simulink model "Powertrain"  (R2020a)
settings: Solver=VariableStepAuto  StartTime=0.0  StopTime=10.0  RelTol=1e-3
values from neighbouring files (symbols this model uses):
  lambda_pm = 0.1194    [MotGenEvDynamicDD.sldd]
undefined symbols (not defined in the file or in its folder): DiscIntNeverNeededParam, Ion, Lithium
libraries: powerlib x12, electricdrivelib x2, powerlib_meascontrol x2, autolibdatasheetbattery x1, simulink x1, autolibmotorctrlr x1, autolibpmsminterior x1, autolibinverter x1
settings Model: Creator=Ricky  LastModifiedBy=Ricky

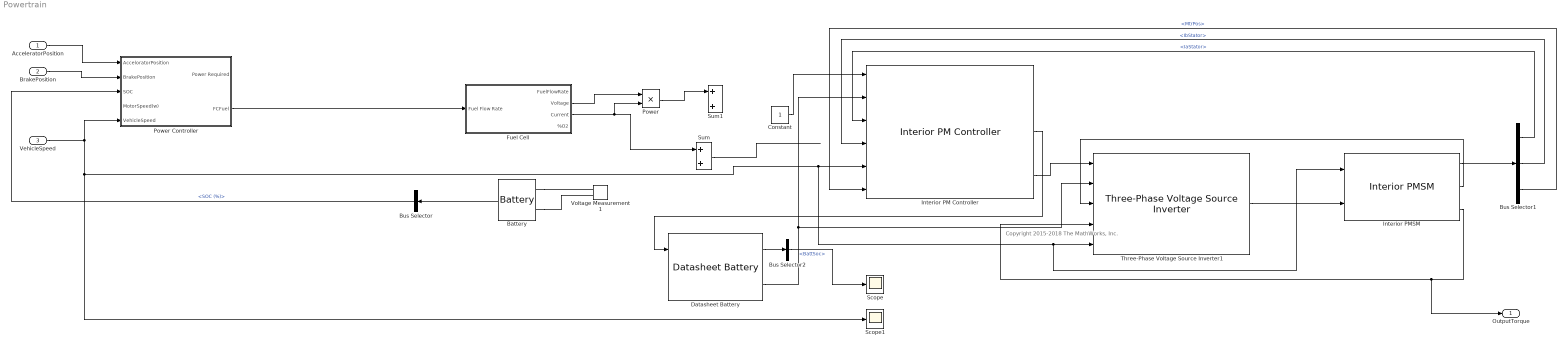
== system Powertrain ==
  note: Copyright 2015-2018 The MathWorks, Inc.
  AcceleratorPosition : Inport
  BrakePosition : Inport  Port=2
  VehicleSpeed : Inport  Port=3
  Battery : electricdrivelib/Extra Sources/Battery  BatType=Lithium-Ion  ShowTempParam=off  ThermalPreset=no  ShowAgeParam=off  NomV=7.2  NomQ=5.4  SOC=100  Batt_Tr=30  PresetModel=on  MaxQ=5.4  MinV=5.4  FullV=8.3807  Dis_rate=2.3478  R=0.013333  Normal_OP=4.8835  expZone="[7.7788      0.2653]"  current=[6.5 13 32.5]  Units=Time  Tci=20  NomT=20  T2=-30  MaxQ2=4.8  FullV2=7.1  Normal_OP2=5.655  expZone2="[6.58           1]"  Rca=0.6  ti=2000  Dp=0  Neq0=0  Tsim=1e6  Ta1=25  Qeol=5.4*0.9  Reol=0.013333*1.2  Char_age=[2.3478, 3]  Dis_age=[2.3478, 10]  N1=1500  N2=10500  N3=1000  N4=1400  Ta2=45  N5=950
  Bus Selector : BusSelector  OutputSignals=SOC (%)
  Bus Selector1 : BusSelector  OutputSignals=IaStator,IbStator,MtrPos
      settings: AttributesFormatString=%<OutputSignals>
  Bus Selector2 : BusSelector  OutputSignals=BattSoc
  Constant : Constant
  Datasheet Battery : autolibdatasheetbattery/Datasheet Battery  CapacityCtrl=Parameter  OutputVlt=Unfiltered  BattChargeMax=100  Em=[2.8 3.228 3.284 3.361 3.408 3.427 3.472 3.477 3.493 3.504 3.516 3.528 3.537 3.545 3.555 3.561 3.566 3.576 3.587 3.589 3.594 3.6 3.608 3.61 3.616 3.619 3.626 3.632 3.637 3.64 3.645 3.646 3.652 3.655 3.658 3.661 3.664 3.668 3.673 3.678 3.68 3.681 3.686 3.692 3.699 3.702 3.705 3.71 3.717 3.723 3.728 3.733 3.735 3.742 3.749 3.755 3.761 3.768 3.773 3.78 3.791 3.798 3.798 3.814 3.818 3.825 3.841 3.846 3.855 3.863 3.877 3.885 3.894 3.907 3.919 3.926 3.935 3.944 3.954 3.964 3.974 3.988 3.998 4.014 4.029 4.034 4.047 4.065 4.074 4.086 4.097 4.131 4.126 4.138 4.15 4.18 4.174 4.187 4.207 4.231 4.221]  CapLUTBp=[0 0.01 0.02 0.03 0.04 0.05 0.06 0.07 0.08 0.09 0.1 0.11 0.12 0.13 0.14 0.15 0.16 0.17 0.18 0.19 0.2 0.21 0.22 0.23 0.24 0.25 0.26 0.27 0.28 0.29 0.3 0.31 0.32 0.33 0.34 0.35 0.36 0.37 0.38 0.39 0.4 0.41 0.42 0.43 0.44 0.45 0.46 0.47 0.48 0.49 0.5 0.51 0.52 0.53 0.54 0.55 0.56 0.57 0.58 0.59 0.6 0.61 0.62 0.63 0.64 0.65 0.66 0.67 0.68 0.69 0.7 0.71 0.72 0.73 0.74 0.75 0.76 0.77 0.78 0.79 0.8 0.81 0.82 0.83 0.84 0.85 0.86 0.87 0.88 0.89 0.9 0.91 0.92 0.93 0.94 0.95 0.96 0.97 0.98 0.99 1]  RInt=[0.008846 0.009319 0.009027 0.00847 0.01032 0.01314;0.006389 0.006554 0.005553 0.005525 0.006043 0.007805;0.004364 0.004101 0.00406 0.003452 0.003846 0.004517;0.002031 0.002563 0.002532 0.00246 0.002716 0.003047;0.001443 0.001825 0.001795 0.001778 0.001924 0.002234;0.0005603 0.0007192 0.0006887 0.0007557 0.0007355 0.001014;0.001028 0.001338 0.001 0.001536 0.001546 0.002789]  BattTempBp=[243.1 253.1 263.1 273.1 283.1 298.1 313.1]  CapSOCBp=[0 0.2 0.4 0.6 0.8 1]  Ns=1  Np=1  BattCapInit=100  Tc=1/1000  Vinit=4.221  RefBlkName='autolibdatasheetbattery/Datasheet Battery'
      settings: SourceProductBaseCode=PW
  Fuel Cell : Subsystem
  Interior PM Controller : autolibmotorctrlr/Interior PM Controller  control_type=Torque Control  Rs=0.02  Ld=1.7e-3  Lq=3.2e-3  lambda_pm=0.2205  PolePairs=4  Mechanical=[0.0027, 4.924e-4, 0]  T_max=60  bp=10  T_mtpa=[0 6.41323967543524 12.8472271930531 19.3221671098192 25.8572437875407 32.4702594835269 39.177408529382 45.9931820911486 52.930379967864 60.0001984561834]  id_mtpa=[0 -0.159333276810563 -0.633258709677809 -1.41005695027301 -2.47173666500257 -3.79592548539108 -5.35786489234899 -7.13217478652462 -9.09420364751938 -11.2209236729158]  iq_mtpa=[0 4.84224935172196 9.66902512748937 14.4660510262181 19.2212063070062 23.9250934510846 28.5711892538614 33.1556572971289 37.6769488702032 42.1353166357157]  idq_limits=[-11.2210468862948 42.1352838229553 43.6038305205566]  EV_current=200  Tst=5e-5  Kp_d=2.1363  Kp_q=4.0212  Ki=25.1327  EV_motion=[20, 4, 0.8]  EV_sf=200  ba=0.40475  Ksa=10.1615  Kisa=41.2325  Ksf=1217.9727  Jcomp=0.0027  Fv=0.0004924  Fs=0  param_loss=Single efficiency measurement  eff=98  w_loss_bp=[0 200 400 600 800 1000]  T_loss_bp=[0 25 50 75 100]  losses_table=[100 100 100 100 100;100 150 200 250 300;100 200 300 400 500;100 250 400 550 700;100 300 500 700 900;100 350 600 850 1100]  w_eff_bp=[200 400 600 800 1000]  T_eff_bp=[25 50 75 100]  efficiency_table=[96.2 98.1 98.7 99;98.1 99 99.4 99.5;98.7 99.4 99.6 99.7;99 99.5 99.7 99.8;99.2 99.6 99.7 99.8]  x_w_bp=[-1000 -800 -600 -400 -200 200 400 600 800 1000]  x_T_bp=[-100 -75 -50 -25 25 50 75 100]  x_losses_mat=[200.400801603196 225.67703109328 200.803212851408 201.612903225806 199.999999999997 200 225 200;160.320641282556 180.541624874624 201.005025125625 202.020202020203 200 200 180 160;180.541624874624 180.722891566267 181.086519114686 197.568389057748 194.999999999999 179.999999999997 180 180;201.005025125625 181.086519114686 202.020202020203 193.67991845056 190 200 179.999999999997 200;202.020202020203 197.568389057748 193.67991845056 197.505197505197 190 190 194.999999999999 200;200 194.999999999999 190 190 197.505197505197 193.67991845056 197.568389057748 202.020202020203;200 179.999999999997 200 190 193.67991845056 202.020202020203 181.086519114686 201.005025125625;180 180 179.999999999997 194.999999999999 197.568389057748 181.086519114686 180.722891566267 180.541624874624;160 180 200 200 202.020202020203 201.005025125625 180.541624874624 160.320641282556;200 225 200 199.999999999997 201.612903225806 200.803212851408 225.67703109328 200.400801603196]  Tsm=5e-4
      settings: SourceProductBaseCode=PW
  Interior PMSM : autolibpmsminterior/Interior PMSM  port_config=Speed  sim_type=Continuous  Ts=0.001  P=4  Rs=.2  Ldq=[3.752e-4 4.148e-4]  KConstText=Permanent flux linkage constant (lambda_pm):  lambda_pm=0.1194  Ke=159.9771  mechanical=[0.0027, 4.924e-4, 0]  idq0=[0 0]  theta_init=0  omega_init=0  KConst=0.1194  lambda_pm_calc=0.1194  Kt=1.323  RefBlkName='autolibpmsminterior/Interior PMSM'  aMode=1
      settings: SourceProductBaseCode=PW,MT,VE,VP
  Power : Product
  Power Controller : Subsystem
  Scope : Scope
  Scope1 : Scope
  Sum : Sum
  Sum1 : Sum
  Three-Phase Voltage Source Inverter1 : autolibinverter/Three-Phase Voltage Source Inverter  InvrtrTmpInpEnbl=off  enable_hdl=off  model_type=Commanded phase voltage  fs=10000  w_eff_bp=[-1000 -500 0 500 1000]  n1=128  T_eff_bp=[-200 -100 0 100 200]  Temp_eff_bp=[213.15 293.15 373.15]  n2=128  ploss_table=[1 0.999 0.989 0.997 0.996;0.995 0.994 0.993 0.992 0.991;0.990 0.989 0.988 0.987 0.986;0.985 0.984 0.983 0.982 0.981;0.980 0.979 0.978 0.977 0.976]  ploss_table_3d=cat(3,0.95*[1 0.999 0.989 0.997 0.996;0.995 0.994 0.993 0.992 0.991;0.990 0.989 0.988 0.987 0.986;0.985 0.984 0.983 0.982 0.981;0.980 0.979 0.978 0.977 0.976],[1 0.999 0.989 0.997 0.996;0.995 0.994 0.993 0.992 0.991;0.990 0.989 0.988 0.987 0.986;0.985 0.984 0.983 0.982 0.981;0.980 0.979 0.978 0.977 0.976],0.92*[1 0.999 0.989 0.997 0.996;0.995 0.994 0.993 0.992 0.991;0.990 0.989 0.988 0.987 0.986;0.985 0.984 0.983 0.982 0.981;0.980 0.979 0.978 0.977 0.976])  preExtrapFlag=off  u1max=1000  u1min=-1000  u2max=200  u2min=-200  intPrec=23  RefBlkName='autolibmappedmotor/Mapped Motor'  CalLossMapData={}  CalLossWithTempMapData={}
      settings: SourceProductBaseCode=PW,MT,VE,VP
  Voltage Measurement1 : powerlib/Measurements/Voltage Measurement  PhasorSimulation=off  OutputType=Complex  PSBequivalent=0
  OutputTorque : Outport
  wires:
  AcceleratorPosition/1 -> Power Controller/1(AcceloratorPosition)
  BrakePosition/1 -> Power Controller/2(BrakePosition)
  VehicleSpeed/1 -> Interior PMSM/1, Three-Phase Voltage Source Inverter1/5, Interior PM Controller/5, Scope1/1, Power Controller/5(VehicleSpeed)
  Interior PMSM/3 -> OutputTorque/1, Three-Phase Voltage Source Inverter1/4
  Power Controller/2(FCFuel) -> Fuel Cell/1(Fuel Flow Rate)
  Sum/1 -> ?
  Battery/1 -> Bus Selector/1
  Bus Selector/1 -> Power Controller/3(SOC)  "<SOC (%)>"
  Fuel Cell/3(Current) -> Power/2, Sum/1
  Fuel Cell/2(Voltage) -> Power/1
  Power/1 -> Sum1/1
  Three-Phase Voltage Source Inverter1/2 -> Interior PMSM/2
  Bus Selector1/3 -> Interior PM Controller/6  "<MtrPos>"
  Bus Selector1/2 -> Interior PM Controller/4  "<IbStator>"
  Interior PMSM/2 -> Three-Phase Voltage Source Inverter1/3
  Bus Selector1/1 -> Interior PM Controller/3  "<IaStator>"
  Interior PMSM/1 -> Bus Selector1/1
  Interior PM Controller/3 -> Three-Phase Voltage Source Inverter1/1
  Datasheet Battery/2 -> Three-Phase Voltage Source Inverter1/2, Interior PM Controller/2
  Constant/1 -> Interior PM Controller/1
  Interior PM Controller/2 -> Datasheet Battery/1
  Datasheet Battery/1 -> Bus Selector2/1
  Bus Selector2/1 -> Scope/1  "<BattSoc>"
  connections:
  Battery/LConn1 -- Voltage Measurement1/LConn1
  Battery/LConn2 -- Voltage Measurement1/LConn2

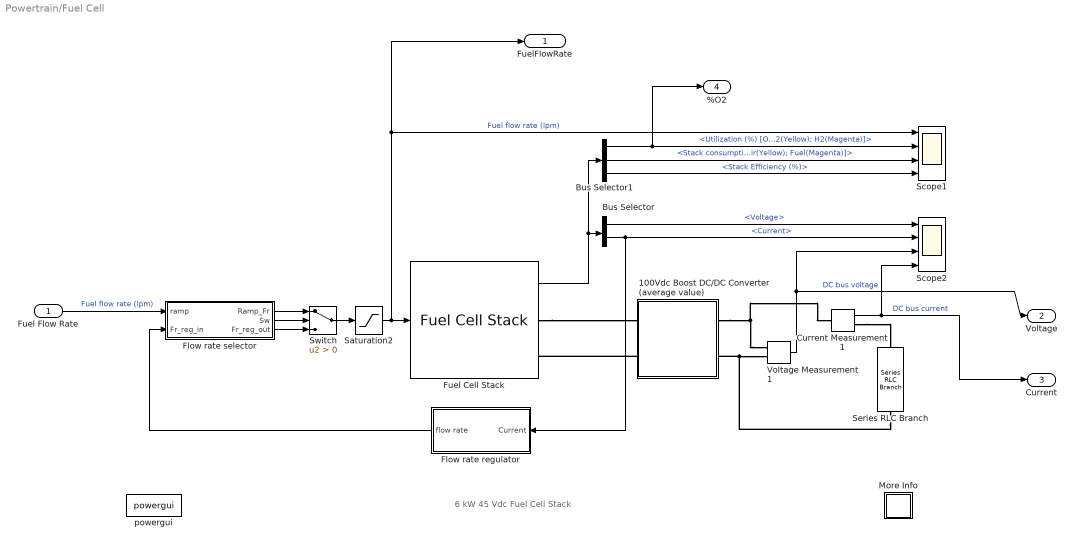
== system Powertrain/Fuel Cell ==
  note: 6 kW 45 Vdc Fuel Cell Stack
  Fuel Flow Rate : Inport
  100Vdc Boost DC/DC Converter (average value) : Subsystem
  Bus Selector : BusSelector  OutputSignals=Voltage,Current
  Bus Selector1 : BusSelector  OutputSignals=Utilization (%) [O2(Yellow); H2(Magenta)],Stack consumption (lpm) [Air(Yellow); Fuel(Magenta)],Stack Efficiency (%)
  Current Measurement1 : powerlib/Measurements/Current Measurement  PhasorSimulation=off  OutputType=Complex  PSBequivalent=0
      settings: SourceProductBaseCode=MT,PS
  Flow rate regulator : Subsystem  mask{Nc=65, Uf_H2=99.56, T=65, Pf=1.5, x=99.95}
      mask prompts: Nc "Number of cells"; Uf_H2 "Nominal Hydrogen utilization (%)"; T "Operating temperature (Celsius)"; Pf "Fuel pressure (bar)"; x "H2 composition (%)"
  Flow rate selector : Subsystem
  Fuel Cell Stack : electricdrivelib/Extra Sources/Fuel Cell Stack  PresetModel=PEMFC - 6 kW - 45 Vdc  FcType=Proton Exchange Membrane (PEM)  Detailed=Detailed  Eoc=[65,63]  NomVI=[133.3,45]  EndVI=[225,37]  Nc=65  n=55  TOp=65  AirFr=300  SuppPress=[1.5,1]  Comp=[99.95,21,1]  SignX=off  SignY=off  FlowRateH2=on  FlowRateAir=off  SystemTemp=off  SystemPH2=off  SystemPAir=off  FCDyn=off  FC_tau=0  Peak_O2=80  V_Under=10
      settings: SourceProductBaseCode=PS
  More Info : Subsystem
      settings: OpenFcn=showdemo(bdroot(gcb))
      mask Display: disp('?')
  Saturation2 : Saturate  UpperLimit=85  LowerLimit=0
  Scope1 : Scope  NumInputPorts=4
  Scope2 : Scope  NumInputPorts=4
  Series RLC Branch : powerlib/Elements/Series RLC Branch  LConnTagsString=__new0  RConnTagsString=__new0  BranchType=RL  Resistance=100*100/6000  Inductance=100*100/6000  SetiL0=off  InitialCurrent=0  Capacitance=1e-6  Setx0=off  InitialVoltage=0  Measurements=None
      settings: SourceProductBaseCode=MT,PS
  Switch : Switch  Criteria=u2 > Threshold
  Voltage Measurement1 : powerlib/Measurements/Voltage Measurement  PhasorSimulation=off  OutputType=Complex  PSBequivalent=0
      settings: SourceProductBaseCode=MT,PS
  powergui : powerlib/powergui  SimulationMode=Continuous  SampleTime=1e-6  frequency=60  Iterations=50  frequencyindice=0  Pbase=100e6  ErrMax=1e-4  UnitsV=kV  UnitsW=MW  buscounter=0  FunctionMessages=off  echomessages=off  EnableUseOfTLC=off  CurrentSourceSwitches=off  DisableSnubberDevices=off  DisableRonSwitches=off  DisableVfSwitches=off  DisplayEquations=off  AutomaticDiscreteSolvers=off  SolverType=Tustin  Interpol=off  ExternalGateDelay=off  methode=off  Ts=0  x0status=blocks  SPID=off  SwTol=0  HookPort=off  NonlinearTolerance=1e-4  nMaxIteration=100  ContinueOnMaxIteration=off  RestoreLinks=warning  ResistiveCurrentMeasurement=off  Frange=[0:2:500]  Ylog=off  Xlog=on  ShowGrid=off  save=off  variable=ZData  structure=0  ZoomFFT=on  StartTime=0.0  cycles=1  DisplayStyle=1  fundamental=60  FreqAxis=off  MaxFrequency=1000  frequencyindicesteady=1  RmsSteady=1  display=off
      settings: SourceProductBaseCode=MT,PS
  FuelFlowRate : Outport
  Voltage : Outport  Port=2
  Current : Outport  Port=3
  %O2 : Outport  Port=4
  wires:
  Bus Selector/1 -> Scope2/1  "<Voltage>"
  Voltage Measurement1/1 -> Scope2/3, Voltage/1  "DC bus voltage"
  Bus Selector/2 -> Scope2/2, Flow rate regulator/1(Current)  "<Current>"
  Bus Selector1/3 -> Scope1/4  "<Stack Efficiency (%)>"
  Saturation2/1 -> Fuel Cell Stack/1, Scope1/1, FuelFlowRate/1  "Fuel flow rate (lpm)"
  Bus Selector1/2 -> Scope1/3  "<Stack consumption (lpm) [Air(Yellow); Fuel(Magenta)]>"
  Flow rate selector/1(Ramp_Fr) -> Switch/1
  Flow rate selector/2(Sw) -> Switch/2
  Bus Selector1/1 -> %O2/1, Scope1/2  "<Utilization (%) [O2(Yellow); H2(Magenta)]>"
  Flow rate regulator/1(flow rate) -> Flow rate selector/2(Fr_reg_in)
  Flow rate selector/3(Fr_reg_out) -> Switch/3
  Fuel Cell Stack/1 -> Bus Selector/1, Bus Selector1/1
  Fuel Flow Rate/1 -> Flow rate selector/1(ramp)  "Fuel flow rate (lpm)"
  Current Measurement1/1 -> Current/1, Scope2/4  "DC bus current"
  Switch/1 -> Saturation2/1
  connections:
  Series RLC Branch/RConn1 -- Voltage Measurement1/LConn2 -- 100Vdc Boost DC/DC Converter (average value)/RConn2
  Voltage Measurement1/LConn1 -- 100Vdc Boost DC/DC Converter (average value)/RConn1 -- Current Measurement1/LConn1
  100Vdc Boost DC/DC Converter (average value)/LConn2 -- Fuel Cell Stack/RConn2
  Current Measurement1/RConn1 -- Series RLC Branch/LConn1
  Fuel Cell Stack/RConn1 -- 100Vdc Boost DC/DC Converter (average value)/LConn1

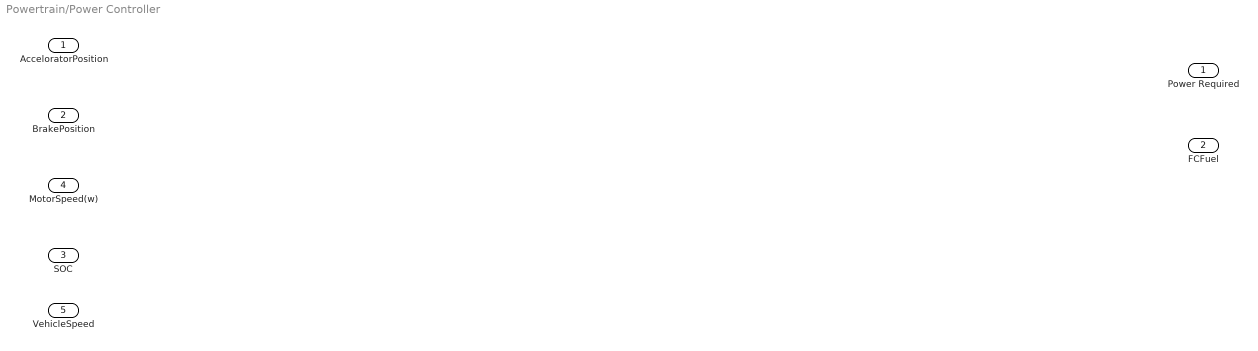
== system Powertrain/Power Controller ==
  AcceloratorPosition : Inport
  BrakePosition : Inport  Port=2
  SOC : Inport  Port=3
  MotorSpeed(w) : Inport  Port=4
  VehicleSpeed : Inport  Port=5
  Power Required : Outport
  FCFuel : Outport  Port=2

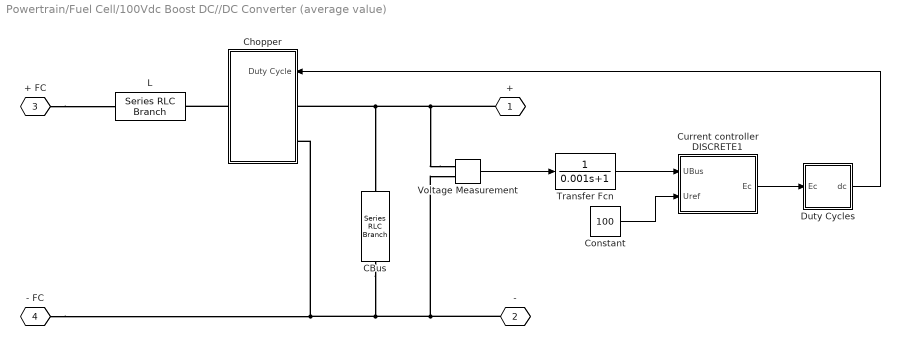
== system Powertrain/Fuel Cell/100Vdc Boost DC//DC Converter (average value) ==
  CBus : powerlib/Elements/Series RLC Branch  LConnTagsString=__new0  RConnTagsString=__new0  BranchType=RC  Resistance=0.2  Inductance=1e-3  SetiL0=off  InitialCurrent=0  Capacitance=7500e-6  Setx0=on  InitialVoltage=100  Measurements=None
      settings: SourceProductBaseCode=MT,PS
  Chopper : Subsystem  mask(SPSdrives Converter){SnubberResistance=10e3, SnubberCapacitance=inf, Ron=1e-3, ForwardVoltages=[1.3,1.3], IGBTParameters=[0,0], converterType=Inverter}
      mask prompts: SnubberResistance "Snubber resistance Rs (Ohms):"; SnubberCapacitance "Snubber capacitance Cs (F):"; Ron "Ron (Ohms):"; ForwardVoltages "Forward voltages [Device Vf(V), Diode Vd (V)]"; IGBTParameters "[Tf(s), Tt(s)]:"; converterType "Converter type:"
      mask help: This model implements an average-value buck converter."Duty Cycle" contains the duty cycle of the internal IGBT device.
      mask TypeOptions converterType: Rectifier | Inverter
      mask Display: plot(0,0,100,100,[39 39 23.8],[71 28 28],[44 56 49.6 56 52.8 56 61 61],[39.2 33.6 32.8 33.6 40.8 33.6 30 12.4],[44 44 44 61 61],[28 71 60 66.4 90],[75 67 83 75 67 83 75 75],[54 42 42 54 54 54 54 66],[61 75 75],[24 24 42],[75 75 61],[66,76,76])
  Constant : Constant  Value=100
  Current controller DISCRETE1 : Subsystem  mask(PI controller){Kp=0.0005, Ki=0.15, Ts=1e-3}
      mask prompts: Kp "Proportional gain (Kp)"; Ki "Integral gain (Ki)"; Ts "Sample time (s) :"
      mask help: Proportional-Integral Speed Controller
      mask Display: plot(0,0,100,100,[35,35,65],[70,30,30],[35,65],[45,60])
  Duty Cycles : Subsystem
  L : powerlib/Elements/Series RLC Branch  LConnTagsString=__new0  RConnTagsString=__new0  BranchType=L  Resistance=0.3  Inductance=500e-6  SetiL0=off  InitialCurrent=0  Capacitance=100e-6  Setx0=off  InitialVoltage=0  Measurements=None
      settings: SourceProductBaseCode=MT,PS
  Transfer Fcn : TransferFcn  Denominator=[0.001 1]
  Voltage Measurement : powerlib/Measurements/Voltage Measurement  PhasorSimulation=off  OutputType=Complex  PSBequivalent=0
      settings: SourceProductBaseCode=MT,PS
  + : PMIOPort  Tag=PMCPort  Side=Right
  - : PMIOPort  Tag=PMCPort  Port=2  Side=Right
  + FC : PMIOPort  Tag=PMCPort  Port=3  Side=Left
  - FC : PMIOPort  Tag=PMCPort  Port=4  Side=Left
  wires:
  Constant/1 -> Current controller DISCRETE1/2(Uref)
  Voltage Measurement/1 -> Transfer Fcn/1
  Duty Cycles/1(dc) -> Chopper/1(Duty Cycle)
  Transfer Fcn/1 -> Current controller DISCRETE1/1(UBus)
  Current controller DISCRETE1/1(Ec) -> Duty Cycles/1(Ec)
  connections:
  - FC/RConn1 -- Voltage Measurement/LConn2 -- -/RConn1 -- CBus/RConn1 -- Chopper/LConn2
  Voltage Measurement/LConn1 -- +/RConn1 -- Chopper/LConn1 -- CBus/LConn1
  Chopper/RConn1 -- L/LConn1
  + FC/RConn1 -- L/RConn1

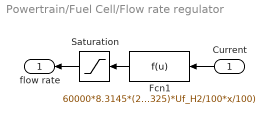
== system Powertrain/Fuel Cell/Flow rate regulator ==
  Current : Inport
  Fcn1 : Fcn  Expr=60000*8.3145*(273+T)*Nc*u(1)/(2*96485*(Pf*101325)*Uf_H2/100*x/100)
  Saturation : Saturate  UpperLimit=inf  LowerLimit=1
  flow rate : Outport  VectorParamsAs1DForOutWhenUnconnected=off
  wires:
  Fcn1/1 -> Saturation/1
  Current/1 -> Fcn1/1
  Saturation/1 -> flow rate/1

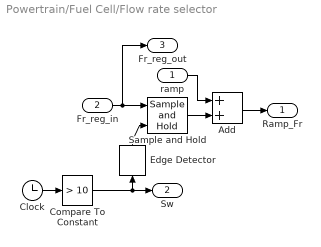
== system Powertrain/Fuel Cell/Flow rate selector ==
  ramp : Inport
  Fr_reg_in : Inport  Port=2
  Add : Sum
  Clock : Clock
  Compare To Constant : simulink/Logic and Bit Operations/Compare To Constant  relop=>  const=10  OutDataTypeStr=boolean
  Edge Detector : powerlib_meascontrol/Logic/Edge Detector  model=Rising  ic=0  Ts=0
      settings: SourceProductBaseCode=MT,PS
  Sample and Hold : powerlib_meascontrol/Additional Components/Sample and Hold  ic=0  Ts=0
      settings: SourceProductBaseCode=MT,PS
  Ramp_Fr : Outport  VectorParamsAs1DForOutWhenUnconnected=off
  Sw : Outport  Port=2  VectorParamsAs1DForOutWhenUnconnected=off
  Fr_reg_out : Outport  Port=3  VectorParamsAs1DForOutWhenUnconnected=off
  wires:
  Clock/1 -> Compare To Constant/1
  Compare To Constant/1 -> Edge Detector/1, Sw/1
  Edge Detector/1 -> Sample and Hold/2
  Sample and Hold/1 -> Add/2
  Fr_reg_in/1 -> Sample and Hold/1, Fr_reg_out/1
  ramp/1 -> Add/1
  Add/1 -> Ramp_Fr/1

== system Powertrain/Fuel Cell/More Info ==

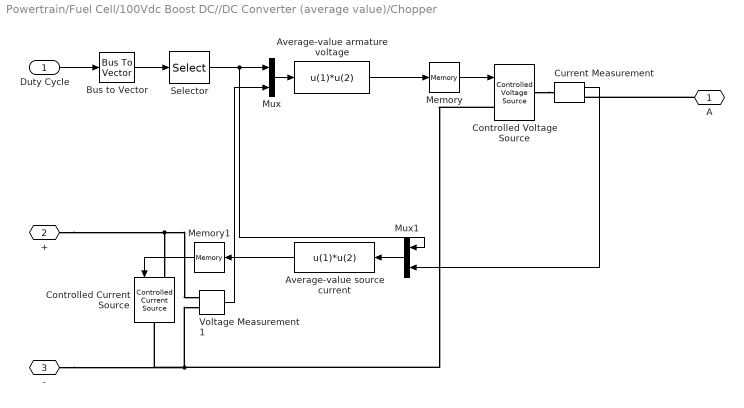
== system Powertrain/Fuel Cell/100Vdc Boost DC//DC Converter (average value)/Chopper ==
  Duty Cycle : Inport
  Average-value armature voltage : Fcn  Expr=u(1)*u(2)
  Average-value source current : Fcn  Expr=u(1)*u(2)
  Bus to Vector : BusToVector
  Controlled Current Source : powerlib/Electrical Sources/Controlled Current Source  Initialize=on  Source_Type=AC  Amplitude=0  Phase=0  Frequency=0  Measurements=None
      settings: SourceProductBaseCode=MT,PS
  Controlled Voltage Source : powerlib/Electrical Sources/Controlled Voltage Source  Initialize=on  Source_Type=AC  Amplitude=0  Phase=0  Frequency=0  Measurements=None
      settings: SourceProductBaseCode=MT,PS
  Current Measurement : powerlib/Measurements/Current Measurement  Tag=PoWeRsYsTeMmEaSuReMeNt  PhasorSimulation=off  OutputType=Magnitude  PSBequivalent=0
      settings: SourceProductBaseCode=MT,PS
  Memory : Memory
  Memory1 : Memory
  Mux : Mux  Inputs=2
  Mux1 : Mux  Inputs=2
  Selector : Selector  InputPortWidth=2  IndexOptions=Index vector (dialog)  Indices=[1]  OutputSizes=1
  Voltage Measurement1 : powerlib/Measurements/Voltage Measurement  Tag=PoWeRsYsTeMmEaSuReMeNt  PhasorSimulation=off  OutputType=Magnitude  PSBequivalent=0
      settings: SourceProductBaseCode=MT,PS
  A : PMIOPort  Side=Right
  + : PMIOPort  Port=2  Side=Left
  - : PMIOPort  Port=3  Side=Left
  wires:
  Selector/1 -> Mux1/1, Mux/1
  Memory1/1 -> Controlled Current Source/1
  Average-value source current/1 -> Memory1/1
  Current Measurement/1 -> Mux1/2
  Mux1/1 -> Average-value source current/1
  Duty Cycle/1 -> Bus to Vector/1
  Voltage Measurement1/1 -> Mux/2
  Mux/1 -> Average-value armature voltage/1
  Average-value armature voltage/1 -> Memory/1
  Memory/1 -> Controlled Voltage Source/1
  Bus to Vector/1 -> Selector/1
  connections:
  A/RConn1 -- Current Measurement/RConn1
  Controlled Voltage Source/RConn1 -- Current Measurement/LConn1
  +/RConn1 -- Voltage Measurement1/LConn1 -- Controlled Current Source/LConn1
  Controlled Voltage Source/LConn1 -- -/RConn1 -- Controlled Current Source/RConn1 -- Voltage Measurement1/LConn2

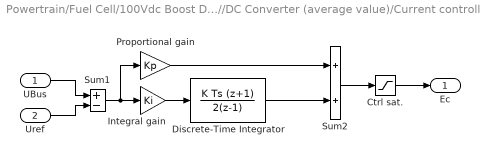
== system Powertrain/Fuel Cell/100Vdc Boost DC//DC Converter (average value)/Current controller DISCRETE1 ==
  UBus : Inport
  Uref : Inport  Port=2
  Ctrl sat. : Saturate  UpperLimit=0.95  LowerLimit=-0.95
  Discrete-Time Integrator : DiscreteIntegrator  IntegratorMethod=Integration: Trapezoidal  SampleTime=Ts  LimitOutput=on  UpperSaturationLimit=0.95  LowerSaturationLimit=-0.95  ICPrevOutput=DiscIntNeverNeededParam  ICPrevScaledInput=DiscIntNeverNeededParam
  Integral gain : Gain  Gain=Ki  SaturateOnIntegerOverflow=on  OutDataTypeStr=Inherit: Same as input  ParamDataTypeStr=Inherit: Same as input
  Proportional gain : Gain  Gain=Kp  SaturateOnIntegerOverflow=on  OutDataTypeStr=Inherit: Same as input  ParamDataTypeStr=Inherit: Same as input
  Sum1 : Sum  Inputs=+-  InputSameDT=on  SaturateOnIntegerOverflow=on  OutDataTypeStr=Inherit: Same as first input
  Sum2 : Sum  InputSameDT=on  SaturateOnIntegerOverflow=on  OutDataTypeStr=Inherit: Same as first input
  Ec : Outport  InitialOutput=0  VectorParamsAs1DForOutWhenUnconnected=off
  wires:
  Ctrl sat./1 -> Ec/1
  Sum2/1 -> Ctrl sat./1
  Discrete-Time Integrator/1 -> Sum2/2
  Uref/1 -> Sum1/2
  UBus/1 -> Sum1/1
  Sum1/1 -> Proportional gain/1, Integral gain/1
  Integral gain/1 -> Discrete-Time Integrator/1
  Proportional gain/1 -> Sum2/1

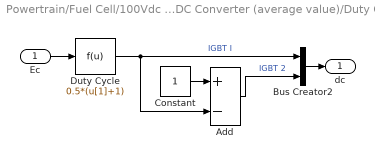
== system Powertrain/Fuel Cell/100Vdc Boost DC//DC Converter (average value)/Duty Cycles ==
  Ec : Inport
  Add : Sum  Inputs=+-
  Bus Creator2 : BusCreator  Inputs=2
  Constant : Constant
  Duty Cycle : Fcn  Expr=0.5*(u[1]+1)
  dc : Outport  VectorParamsAs1DForOutWhenUnconnected=off
  wires:
  Bus Creator2/1 -> dc/1
  Ec/1 -> Duty Cycle/1
  Constant/1 -> Add/1
  Add/1 -> Bus Creator2/2  "IGBT 2"
  Duty Cycle/1 -> Bus Creator2/1, Add/2  "IGBT I"
